simulink model "Second_Order_System"  (Simulink 7.1)
settings: Solver=ode45  StartTime=0.0  StopTime=Tf  MaxStep=1e-5  RelTol=1e-3
values from neighbouring files (symbols this model uses):
  Amp = x(end)    [second_order_driver.m]
  K = 1.5    [second_order_driver.m]
  omega_n = 10.0    (= 10)    [second_order_driver.m]
  zeta = 0.05    [second_order_driver.m]
settings Model: Creator=throne  LastModifiedBy=throne

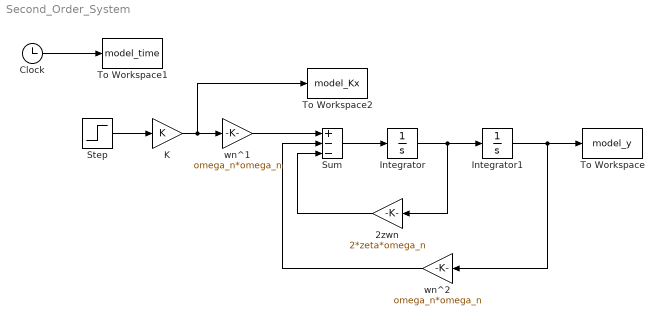
== system Second_Order_System ==
  2zwn : Gain  Orientation=left  Gain=2*zeta*omega_n  ParameterDataType=sfix(16)  ParameterScaling=2^0  OutDataType=sfix(16)  OutScaling=2^0
  Clock : Clock
      settings: Decimation=10
  Integrator : Integrator
  Integrator1 : Integrator
  K : Gain  Gain=K  ParameterDataType=sfix(16)  ParameterScaling=2^0  OutDataType=sfix(16)  OutScaling=2^0
  Step : Step  Time=0  After=Amp  SampleTime=0
  Sum : Sum  Inputs=|+|-|-|  OutDataType=sfix(16)  OutScaling=2^0
  To Workspace : ToWorkspace  VariableName=model_y  SampleTime=-1  SaveFormat=Array
  To Workspace1 : ToWorkspace  VariableName=model_time  SampleTime=-1  SaveFormat=Array
  To Workspace2 : ToWorkspace  VariableName=model_Kx  SampleTime=-1  SaveFormat=Array
  wn^1 : Gain  Gain=omega_n*omega_n  ParameterDataType=sfix(16)  ParameterScaling=2^0  OutDataType=sfix(16)  OutScaling=2^0
  wn^2 : Gain  Orientation=left  Gain=omega_n*omega_n  ParameterDataType=sfix(16)  ParameterScaling=2^0  OutDataType=sfix(16)  OutScaling=2^0
  wires:
  Sum/1 -> Integrator/1
  Clock/1 -> To Workspace1/1
  Integrator/1 -> Integrator1/1, 2zwn/1
  Integrator1/1 -> To Workspace/1, wn^2/1
  2zwn/1 -> Sum/3
  wn^2/1 -> Sum/2
  Step/1 -> K/1
  wn^1/1 -> Sum/1
  K/1 -> wn^1/1, To Workspace2/1
